simulink model "combined"  (R2023a)
settings: Solver=VariableStepAuto  StartTime=0.0  StopTime=10.0  RelTol=1e-3
libraries: embmathops x1
settings Model: Creator=yaboi  LastModifiedBy=yaboi

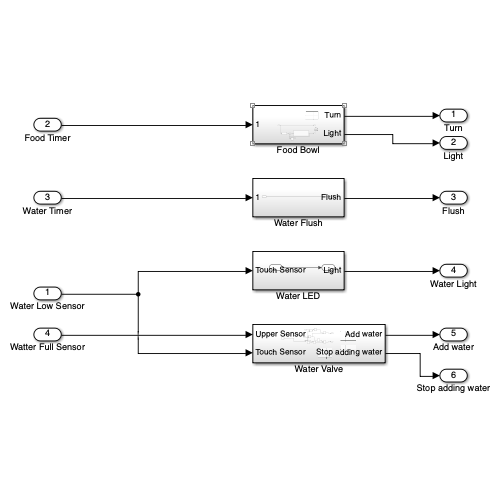
[thumbnail: Simulink's stored preview of the top-level diagram]
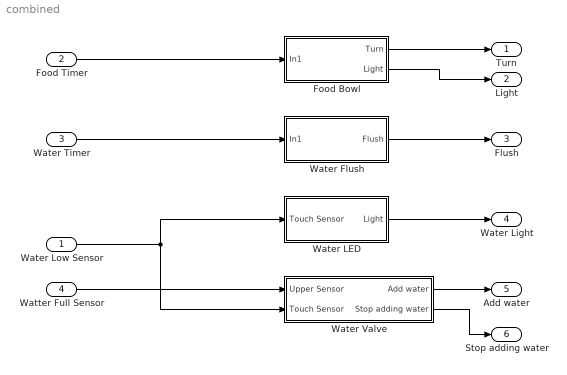
== system combined ==
  Water Low Sensor : Inport
  Food Timer : Inport  Port=2
  Water Timer : Inport  Port=3
  Watter Full Sensor : Inport  Port=4
  Food Bowl : Subsystem
  Water Flush : Subsystem
  Water LED : Subsystem
  Water Valve : Subsystem
  Turn : Outport
  Light : Outport  Port=2
  Flush : Outport  Port=3
  Water Light : Outport  Port=4
  Add water : Outport  Port=5
  Stop adding water : Outport  Port=6
  wires:
  Water Low Sensor/1 -> Water Valve/2(Touch Sensor), Water LED/1(Touch Sensor)
  Food Timer/1 -> Food Bowl/1(In1)
  Water Timer/1 -> Water Flush/1(In1)
  Watter Full Sensor/1 -> Water Valve/1(Upper Sensor)
  Food Bowl/1(Turn) -> Turn/1
  Food Bowl/2(Light) -> Light/1
  Water Flush/1(Flush) -> Flush/1
  Water LED/1(Light) -> Water Light/1
  Water Valve/1(Add water) -> Add water/1
  Water Valve/2(Stop adding water) -> Stop adding water/1

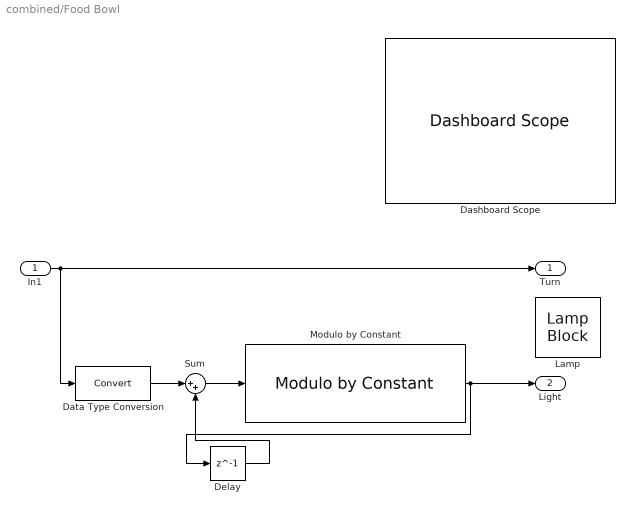
== system combined/Food Bowl ==
  In1 : Inport
  Dashboard Scope : DashboardScope
  Data Type Conversion : DataTypeConversion  OutMin=0  OutMax=1  ConvertRealWorld=Stored Integer (SI)  RndMeth=Nearest  SaturateOnIntegerOverflow=off
  Delay : Delay  DelayLength=1  InitialCondition=0
  Lamp : LampBlock  LabelPosition=Hide
  Modulo by Constant : embmathops/Modulo by Constant  Denominator=6  SimulateUsing=Code generation
      settings: LibrarySourceBlock=embeddedMathLib/Modulo by Constant
  Sum : Sum  Inputs=|++
  Turn : Outport
  Light : Outport  Port=2
  wires:
  In1/1 -> Data Type Conversion/1, Turn/1
  Modulo by Constant/1 -> Delay/1, Light/1
  Sum/1 -> Modulo by Constant/1
  Data Type Conversion/1 -> Sum/1
  Delay/1 -> Sum/2

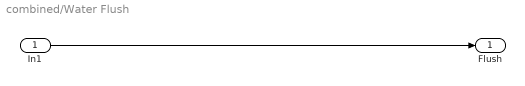
== system combined/Water Flush ==
  In1 : Inport
  Flush : Outport
  wires:
  In1/1 -> Flush/1

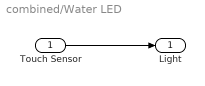
== system combined/Water LED ==
  Touch Sensor : Inport
  Light : Outport
  wires:
  Touch Sensor/1 -> Light/1

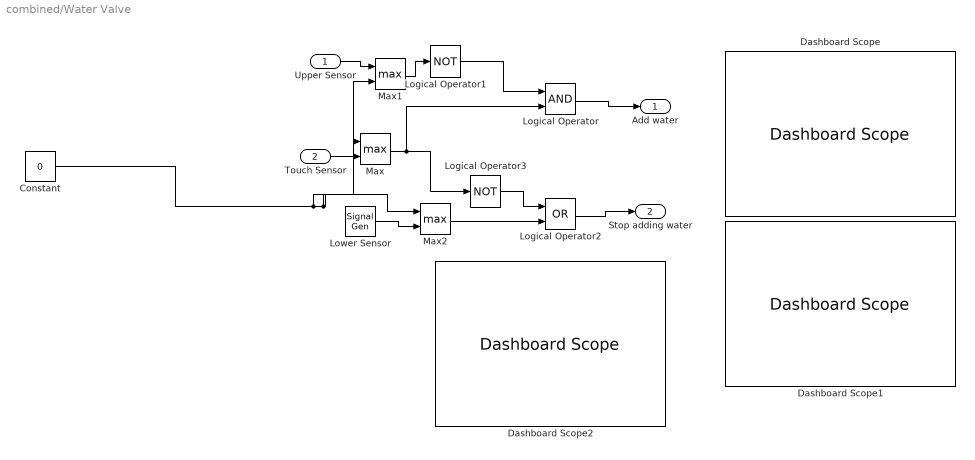
== system combined/Water Valve ==
  Upper Sensor : Inport
  Touch Sensor : Inport  Port=2
  Constant : Constant  Value=0
  Dashboard Scope : DashboardScope
  Dashboard Scope1 : DashboardScope
  Dashboard Scope2 : DashboardScope
  Logical Operator : Logic  AllPortsSameDT=off  OutDataTypeStr=boolean
  Logical Operator1 : Logic  Operator=NOT  AllPortsSameDT=off  OutDataTypeStr=boolean
  Logical Operator2 : Logic  Operator=OR  AllPortsSameDT=off  OutDataTypeStr=boolean
  Logical Operator3 : Logic  Operator=NOT  AllPortsSameDT=off  OutDataTypeStr=boolean
  Lower Sensor : SignalGenerator  WaveForm=square  Frequency=2  Units=rad/sec
  Max : MinMax  Function=max  Inputs=2
  Max1 : MinMax  Function=max  Inputs=2
  Max2 : MinMax  Function=max  Inputs=2
  Add water : Outport
  Stop adding water : Outport  Port=2
  wires:
  Lower Sensor/1 -> Max2/2
  Logical Operator1/1 -> Logical Operator/1
  Upper Sensor/1 -> Max1/1
  Constant/1 -> Max2/1, Max1/2, Max/1
  Logical Operator2/1 -> Stop adding water/1
  Logical Operator3/1 -> Logical Operator2/1
  Touch Sensor/1 -> Max/2
  Logical Operator/1 -> Add water/1
  Max1/1 -> Logical Operator1/1
  Max/1 -> Logical Operator/2, Logical Operator3/1
  Max2/1 -> Logical Operator2/2
